simulink model "hoverSim_pid"  (R2025b)
settings: Solver=ode45  StartTime=0.0  StopTime=30  RelTol=1e-3  AbsTol=1e-3  EnableMultiTasking=on
values from neighbouring files (symbols this model uses):
  A = [0 0 0 1 0 0 ... (first row only)    [setupHover.m]    (also in setupVerdier.mat = [0 0 0 0 0 0 0 0 0 0 0 0 ... (36 elements, 6x6)])
  B = [0     0     0     0 ... (first row only)    [setupHover.m]    (also in setupVerdier.mat = [0 0 0 -0.0325954333483 0.423483129605 0 0 0 0 -0.0325954333)
  C = [1 0 0 0 0 0 ... (first row only)    [setupHover.m]    (also in setupVerdier.mat = [1 0 0 0 1 0 0 0 1 0 0 0 ... (18 elements, 3x6)])
  CMD_RATE_LIMIT = 60 * pi/180    (= 1.0471975512)    [setupHover.m]    (also in setupVerdier.mat)
  D = zeros(3,4)    [setupHover.m]    (also in setupVerdier.mat = [0  0  0  0; 0  0  0  0; 0  0  0  0])
  K = [ 1  1  0 ... (first row only)    [setupHover.m]    (also in setupVerdier.mat = [-111.8 -111.8 111.8 111.8 132.3 -132.3 0 0 0 0 132.3 -132.3)
  V_bias = 2.0    (= 2)    [setupHover.m]    (also in setupVerdier.mat)
  VMAX_AMP = 24    [setupHover.m]    (also in setupVerdier.mat)
  wcf = 2 * pi * 20    (= 125.663706144)    [setupHover.m]    (also in setupVerdier.mat)
  zetaf = 0.6    [setupHover.m]    (also in setupVerdier.mat)
undefined symbols (not defined in the file or in its folder): X, Y, Z
libraries: sm_lib x30, simulink_extras x19, nesl_utility x4, simulink x1
(part 1 of 2)
settings Model: Creator=2922887  LastModifiedBy=oleruus
settings SolverCC: AutoScaleAbsTol=off  AlgebraicLoopSolver=TrustRegion
settings DataIOCC: LimitDataPoints=on  MaxDataPoints=10000
settings OptimizationCC: LifeSpan=inf
settings DebuggingCC: UnconnectedInputMsg=warning  UnconnectedOutputMsg=warning  UnconnectedLineMsg=warning  AllowSymbolicDim=off  SFUnexpectedBacktrackingDiag=warning  SFNoUnconditionalDefaultTransitionDiag=warning  SFExecutionAtInitializationDiag=none  ArithmeticOperatorsInVariantConditions=warning
settings ModelReferenceCC: EnableRefExpFcnMdlSchedulingChecks=on
settings SFSimCC: SimUseLocalCustomCode=off  CustomCodeUndefinedFunction=UseInterfaceOnly
settings RTWCC: RTWUseLocalCustomCode=off  GPUComputeCapability=3.5  DLArmComputeVersion=19.05
settings CodeAppCC: StateflowObjectComments=on
settings GRTTargetCC: TargetLangStandard=C89/C90 (ANSI)
settings ConfigComp: CovMetricSettings=dw  CovSaveCumulativeToWorkspaceVar=on  CovSaveSingleToWorkspaceVar=on  CovExternalEMLEnable=off  CovSFcnEnable=off
settings SimscapeCC: SimscapeLogType=all  SimscapeLogSimulationStatistics=on  SimscapeLogDataHistory=10000.0
settings ExplorerConfigSet: InternalSimMechanicsExplorerSettings="<ExplorerConfiguration><canonicalview>default</canonicalview><AnimationSetting><BasePlaybackSpeed>1.0</BasePlaybackSpeed><PlaybackSpeedFactor>1.0</PlaybackSpeedFactor></AnimationSetting><TilePanel><TileInfo><Tiles Columns=\"1\" Count=\"1\" Rows=\"1\"><Column Weight=\"1\"/><Row Weight=\"1\"/><Tile Height=\"1\" Width=\"1\" X=\"0\" Y=\"0\"/></Tiles></TileInfo><SceneInfo><SceneViewer><BGColor><R>1</R><G>1</G><B>1</B></BGColor><Camera><DoPerspective>off</DoPerspective><Position><X>-0.474872206876914782</X><Y>-0.66192885214412267</Y><Z>0.674687949495536343</Z></Position><Center><X>0.0282179779907451508</X><Y>0.0797842513243843532</Y><Z>0.231109390462924141</Z></Center><Up><X>0.245225672410919443</X><Y>0.369652493337906174</Y><Z>0.896226201223598418</Z></Up><ViewLimDist>1</ViewLimDist><YLim>0.878174162375433998</YLim><XLim>0.626410921284865863</XLim></Camera></SceneViewer></SceneInfo></TilePanel><MechEditorPanel><Cameras/><GfxPanelCameraMap/><VideoCreator><PlaybackSpeedRatio>1.0</PlaybackSpeedRatio><FrameRate>30</FrameRate><VideoFormat>Motion JPEG AVI</VideoFormat><FrameSize>auto</FrameSize></VideoCreator></MechEditorPanel></ExplorerConfiguration>"

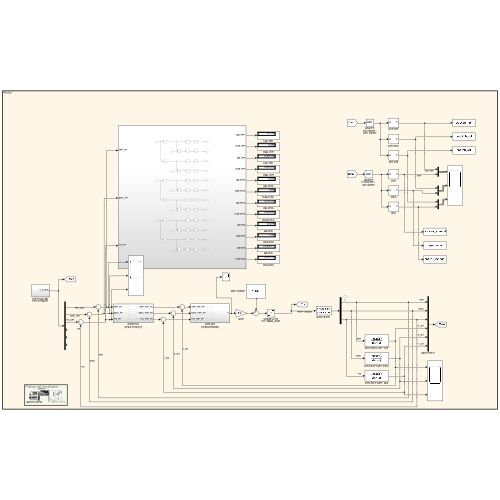
[thumbnail: Simulink's stored preview of the top-level diagram]
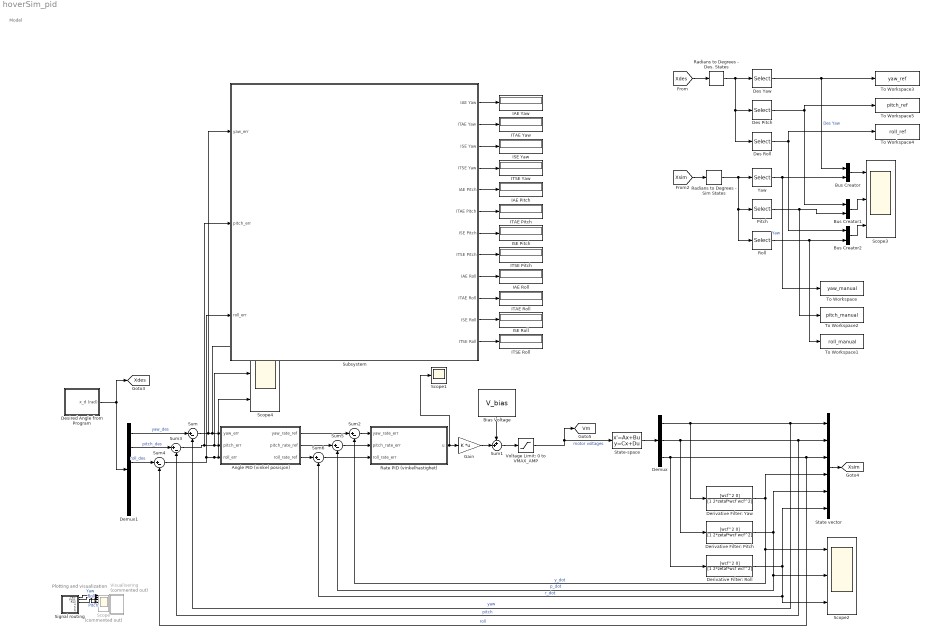
== system hoverSim_pid ==
  note: Plotting and visualization
  note: Model
  Angle PID (vinkel posisjon) : Subsystem
  Bias Voltage : Constant  Value=V_bias
  Bus Creator : BusCreator  Inputs=2
  Bus Creator1 : BusCreator  Inputs=2
  Bus Creator2 : BusCreator  Inputs=2
  Demux : Demux  Outputs=3
  Demux1 : Demux  Outputs=6
  Derivative Filter: Pitch : TransferFcn  Numerator=[wcf^2 0]  Denominator=[1 2*zetaf*wcf wcf^2]
  Derivative Filter: Roll : TransferFcn  Numerator=[wcf^2 0]  Denominator=[1 2*zetaf*wcf wcf^2]
  Derivative Filter: Yaw : TransferFcn  Numerator=[wcf^2 0]  Denominator=[1 2*zetaf*wcf wcf^2]
  Des Pitch : Selector  InputPortWidth=6  IndexOptions=Index vector (dialog)  Indices=2  OutputSizes=1
  Des Roll : Selector  InputPortWidth=6  IndexOptions=Index vector (dialog)  Indices=3  OutputSizes=1
  Des Yaw : Selector  InputPortWidth=6  IndexOptions=Index vector (dialog)  Indices=1  OutputSizes=1
  Desired Angle from Program : Subsystem
  Gain : Gain  Gain=K  Multiplication=Matrix(K*u)
  IAE Pitch : Display
  IAE Roll : Display
  IAE Yaw : Display
  ISE Pitch : Display
  ISE Roll : Display
  ISE Yaw : Display
  ITAE Pitch : Display
  ITAE Roll : Display
  ITAE Yaw : Display
  ITSE Pitch : Display
  ITSE Roll : Display
  ITSE Yaw : Display
  Pitch : Selector  InputPortWidth=6  IndexOptions=Index vector (dialog)  Indices=2  OutputSizes=1
  Radians to Degrees - Des. States : simulink_extras/Transformations/Radians to Degrees
  Radians to Degrees - Sim States : simulink_extras/Transformations/Radians to Degrees
  Rate PID (vinkelhastighet) : Subsystem
  Roll : Selector  InputPortWidth=6  IndexOptions=Index vector (dialog)  Indices=3  OutputSizes=1
  Scope : Scope  Commented=on  NumInputPorts=8
      settings: TimeSpan=30  Title=Yaw angle  ActiveDisplayYMinimum=-0.13556328685878161  ActiveDisplayYMaximum=1.2200695817290348  YLabel=deg  DataLoggingMaxPoints=10000  DataLoggingVariableName=simulationOutput
  Scope1 : Scope
      settings: ActiveDisplayYMinimum=-981.01331682218438  ActiveDisplayYMaximum=1141.4224649805096
  Scope2 : Scope  NumInputPorts=3
      settings: ActiveDisplayYMinimum=-0.50081800652745567  ActiveDisplayYMaximum=0.50362688913760034
  Scope3 : Scope  NumInputPorts=3
      settings: ActiveDisplayString=3  Title=Roll  ActiveDisplayYMinimum=-0.12798954340312932  ActiveDisplayYMaximum=1.1519058906281641  YLabel=Deg  DataLoggingVariableName=ScopeData2
  Scope4 : Scope  NumInputPorts=3
      settings: ActiveDisplayString=3  Title=Roll  ActiveDisplayYMinimum=-0.0024405494877172713  ActiveDisplayYMaximum=0.017790755348184792  YLabel=Deg  DataLoggingVariableName=ScopeData3
  Signal routing : Subsystem
  State vector : Mux  Inputs=6
  State-space : StateSpace  A=A  B=B  C=C  D=D  InitialCondition=0
  Subsystem : Subsystem
  Sum{,2..6} (6 alike) : Sum  Inputs=|+-
  Sum1 : Sum  Inputs=++|
  To Workspace : ToWorkspace  VariableName=yaw_manual  SaveFormat=Timeseries  SampleTime=-1
  To Workspace1 : ToWorkspace  VariableName=roll_manual  SaveFormat=Timeseries  SampleTime=-1
  To Workspace2 : ToWorkspace  VariableName=pitch_manual  SaveFormat=Timeseries  SampleTime=-1
  To Workspace3 : ToWorkspace  VariableName=yaw_ref  SaveFormat=Timeseries  SampleTime=-1
  To Workspace4 : ToWorkspace  VariableName=roll_ref  SaveFormat=Timeseries  SampleTime=-1
  To Workspace5 : ToWorkspace  VariableName=pitch_ref  SaveFormat=Timeseries  SampleTime=-1
  Visualisering : Subsystem  Commented=on  mask{visualization=Visualization off, PacingRate=1}
      mask prompts: PacingRate "Simulation ratio (1:x) time vs real time"
      mask TypeOptions visualization: Visualization  on | Visualization off
      mask Callback visualization:
      | if get_param(append(bdroot,'/Visualisering'),'visualization') == 'Visualization  on'
      |    set_param(bdroot,'EnablePacing','on')
      | elseif get_param(append(bdroot,'/Visualisering'),'visualization') == 'Visualization off'
      |    set_param(bdroot,'EnablePacing','off')
      | end
      mask Callback PacingRate:
      | temp_param = str2num(get_param(append(bdroot,'/Visualisering'),'PacingRate'));
      | if temp_param >= 0.003 && temp_param < 0.0078
      |     set_param(bdroot,'PacingRate','0.0039')
      |     set_param(append(bdroot,'/Visualisering'),'PacingRate','0.0039')
      | elseif temp_param >= 0.0078 && temp_param < 0.0156
      |     set_param(bdroot,'PacingRate','0.0078')
      |     set_param(append(bdroot,'/Visualisering'),'PacingRate','0.0078')
      | elseif temp_param >= 0.0156 && temp_param < 0.0313
      |     set_param(bdroot,'PacingRate','0.0156')
      |     set_param(append(bdroot,'/Visualisering'),'PacingRate','0.0156')
      | elseif temp_param >= 0.0313 && temp_param < 0.0625
      |     set_param(bdroot,'PacingRate','0.0313')
      |     set_param(append(bdroot,'/Visualisering'),'PacingRate','0.0313')
      | elseif temp_param >= 0.0625 && temp_param < 0.1250
      |     set_param(bdroot,'PacingRate','0.0625')
      |     set_param(append(bdroot,'/Visualisering'),'PacingRate','0.0625')
      | elseif temp_param >= 0.1250 && temp_param < 0.2500
      |     set_param(bdroot,'PacingRate','0.1250')
      |     set_param(append(bdroot,'/Visualisering'),'PacingRate','0.1250')
      | elseif temp_param >= 0.2500 && temp_param < 0.5000
      |     set_param(bdroot, 'PacingRate','0.2500')
      |     set_param(append(bdroot,'/Visualisering'),'PacingRate','0.2500')
      | elseif temp_param >= 0.5000 && temp_param < 1
      |     set_param(bdroot, 'PacingRate','0.5000')
      |     set_param(append(bdroot,'/Visualisering'),'PacingRate','0.5000')
      | elseif temp_param >= 1 && temp_param < 2
      |     set_param(bdroot, 'PacingRate','1')
      |     set_param(append(bdroot,'/Visualisering'),'PacingRate','1')
      | elseif temp_param >= 2 && temp_param < 4
      |     set_param(bdroot, 'PacingRate','2')
      |     set_param(append(bdroot,'/Visualisering'),'PacingRate','2')
      | elseif temp_param >= 4 && temp_param < 8
      |     set_param(bdroot, 'PacingRate','4')
      |     set_param(append(bdroot,'/Visualisering'),'PacingRate','4')
      | elseif temp_param >= 8 && temp_param < 16
      |     set_param(bdroot, 'PacingRate','8')
      |     set_param(append(bdroot,'/Visualisering'),'PacingRate','8')
      | elseif temp_param >= 16 && temp_param < 32
      |     set_param(bdroot, 'PacingRate','16')
      |     set_param(append(bdroot,'/Visualisering'),'PacingRate','16')
      | elseif temp_param >= 32 && temp_param < 64
      |     set_param(bdroot, 'PacingRate','32')
      |     set_param(append(bdroot,'/Visualisering'),'PacingRate','32')
      | elseif temp_param >= 64 && temp_param < 128
      |     set_param(bdroot, 'PacingRate','64')
      |     set_param(append(bdroot,'/Visualisering'),'PacingRate','64')
      | elseif temp_param >= 128 && temp_param < 256
      |     set_param(bdroot, 'PacingRate','128')
      |     set_param(append(bdroot,'/Visualisering'),'PacingRate','128')
      | elseif temp_param >= 256
      |     set_param(bdroot, 'PacingRate','256')
      |     set_param(append(bdroot,'/Visualisering'),'PacingRate','256')
      | end
      mask DialogControl Control2 Prompt: For a 1:1 relation between the visualization model and the plotted data, the simulation ratio in this box should match the ratio in the Mechanics Explorer.
      mask DialogControl x256x Prompt: 0.0039 = 1/256x
      mask DialogControl x128x Prompt: 0.0078 = 1/128x
      mask DialogControl x64x Prompt: 0.0156 = 1/64x
      mask DialogControl x32x Prompt: 0.0313 = 1/32x
      mask DialogControl x16x Prompt: 0.0625 = 1/16x
      mask DialogControl x8x Prompt: 0.1250 = 1/8x
      mask DialogControl x4x Prompt: 0.2500 = 1/4x
      mask DialogControl x2x Prompt: 0.5000 = 1/2x
      mask Display: image('$imagefile'); % Use "Edit Image" on toolstrip to change.
  Voltage Limit: 0 to VMAX_AMP : Saturate  UpperLimit=VMAX_AMP  LowerLimit=0  LinearizeAsGain=off
  Yaw : Selector  InputPortWidth=6  IndexOptions=Index vector (dialog)  Indices=1  OutputSizes=1
  tag scope: Vm=global, Xdes=global, Xsim=global
  wires:
  Gain/1 -> Sum1/2
  Voltage Limit: 0 to VMAX_AMP/1 -> [Vm], State-space/1  "motor voltages"
  Derivative Filter: Roll/1 -> Scope2/3, Sum6/2, State vector/6  "r_dot"
  Derivative Filter: Yaw/1 -> Sum2/2, Scope2/1, State vector/4  "y_dot"
  State-space/1 -> Demux/1
  State vector/1 -> [Xsim]
  Demux/1 -> Derivative Filter: Yaw/1, Sum/2, State vector/1  "yaw"
  Sum1/1 -> Voltage Limit: 0 to VMAX_AMP/1
  Bias Voltage/1 -> Sum1/1
  Demux/2 -> Derivative Filter: Pitch/1, State vector/2, Sum3/2  "pitch"
  Derivative Filter: Pitch/1 -> Scope2/2, Sum5/2, State vector/5  "p_dot"
  Demux/3 -> State vector/3, Sum4/2, Derivative Filter: Roll/1  "roll"
  Signal routing/1(Yaw) -> Scope/1  "Yaw"
  Signal routing/2(Pitch) -> Scope/4, Scope/2  "Pitch"
  Signal routing/3(Roll) -> Scope/3  "Roll"
  Desired Angle from Program/1(x_d (rad)) -> Demux1/1, [Xdes]
  Sum2/1 -> Rate PID (vinkelhastighet)/1(yaw_rate_err)
  Demux1/1 -> Sum/1  "yaw_des"
  Sum/1 -> Subsystem/1(yaw_err), Scope4/1, Angle PID (vinkel posisjon)/1(yaw_err)
  Demux1/2 -> Sum3/1  "pitch_des"
  Demux1/3 -> Sum4/1  "roll_des"
  Sum3/1 -> Subsystem/2(pitch_err), Scope4/2, Angle PID (vinkel posisjon)/2(pitch_err)
  Sum4/1 -> Subsystem/3(roll_err), Scope4/3, Angle PID (vinkel posisjon)/3(roll_err)
  Rate PID (vinkelhastighet)/1(u) -> Scope1/1, Gain/1
  Sum5/1 -> Rate PID (vinkelhastighet)/2(pitch_rate_err)
  Sum6/1 -> Rate PID (vinkelhastighet)/3(roll_rate_err)
  Angle PID (vinkel posisjon)/1(yaw_rate_ref) -> Sum2/1
  Angle PID (vinkel posisjon)/2(pitch_rate_ref) -> Sum5/1
  Angle PID (vinkel posisjon)/3(roll_rate_ref) -> Sum6/1
  Des Pitch/1 -> Bus Creator1/1, To Workspace5/1
  Pitch/1 -> To Workspace2/1, Bus Creator1/2
  Yaw/1 -> To Workspace/1, Bus Creator/2  "Yaw"
  Des Roll/1 -> Bus Creator2/1, To Workspace4/1
  Des Yaw/1 -> Bus Creator/1, To Workspace3/1  "Des Yaw"
  Radians to Degrees - Sim States/1 -> Roll/1, Pitch/1, Yaw/1
  [Xsim] -> Radians to Degrees - Sim States/1
  [Xdes] -> Radians to Degrees - Des. States/1
  Radians to Degrees - Des. States/1 -> Des Roll/1, Des Pitch/1, Des Yaw/1
  Roll/1 -> To Workspace1/1, Bus Creator2/2
  Bus Creator/1 -> Scope3/1
  Bus Creator1/1 -> Scope3/2
  Bus Creator2/1 -> Scope3/3
  Subsystem/10(ITAE Roll) -> ITAE Roll/1
  Subsystem/9(IAE Roll) -> IAE Roll/1
  Subsystem/1("IAE Yaw ") -> IAE Yaw/1
  Subsystem/2(ITAE Yaw) -> ITAE Yaw/1
  Subsystem/5(IAE Pitch) -> IAE Pitch/1
  Subsystem/6(ITAE Pitch) -> ITAE Pitch/1
  Subsystem/3(ISE Yaw) -> ISE Yaw/1
  Subsystem/4(ITSE Yaw) -> ITSE Yaw/1
  Subsystem/7(ISE Pitch) -> ISE Pitch/1
  Subsystem/8(ITSE Pitch) -> ITSE Pitch/1
  Subsystem/11(ISE Roll) -> ISE Roll/1
  Subsystem/12(ITSE Roll) -> ITSE Roll/1

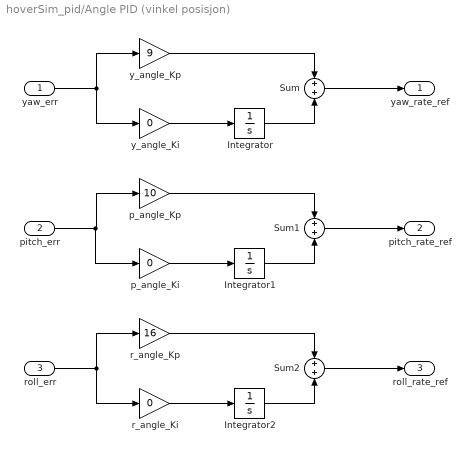
== system hoverSim_pid/Angle PID (vinkel posisjon) ==
  yaw_err : Inport
  pitch_err : Inport  Port=2
  roll_err : Inport  Port=3
  Integrator : Integrator
  Integrator1 : Integrator
  Integrator2 : Integrator
  Sum : Sum  Inputs=+|+
  Sum1 : Sum  Inputs=+|+
  Sum2 : Sum  Inputs=+|+
  p_angle_Ki : Gain  Gain=0
  p_angle_Kp : Gain  Gain=10
  r_angle_Ki : Gain  Gain=0
  r_angle_Kp : Gain  Gain=16
  y_angle_Ki : Gain  Gain=0
  y_angle_Kp : Gain  Gain=9
  yaw_rate_ref : Outport
  pitch_rate_ref : Outport  Port=2
  roll_rate_ref : Outport  Port=3
  wires:
  Sum/1 -> yaw_rate_ref/1
  pitch_err/1 -> p_angle_Ki/1, p_angle_Kp/1
  p_angle_Ki/1 -> Integrator1/1
  Integrator1/1 -> Sum1/2
  p_angle_Kp/1 -> Sum1/1
  y_angle_Kp/1 -> Sum/1
  Integrator/1 -> Sum/2
  y_angle_Ki/1 -> Integrator/1
  yaw_err/1 -> y_angle_Ki/1, y_angle_Kp/1
  Sum1/1 -> pitch_rate_ref/1
  roll_err/1 -> r_angle_Kp/1, r_angle_Ki/1
  r_angle_Kp/1 -> Sum2/1
  r_angle_Ki/1 -> Integrator2/1
  Integrator2/1 -> Sum2/2
  Sum2/1 -> roll_rate_ref/1

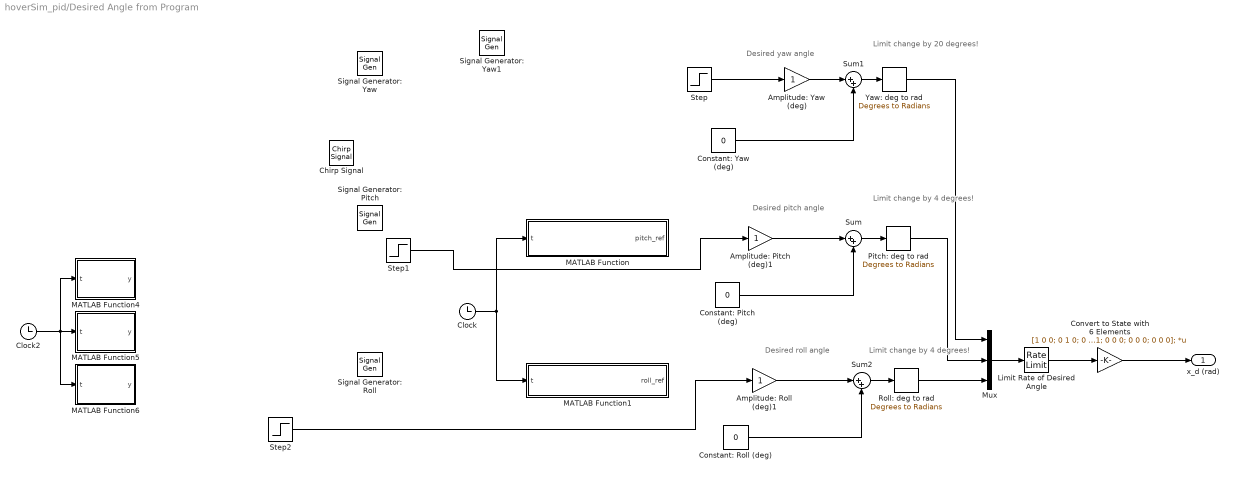
== system hoverSim_pid/Desired Angle from Program ==
  note: Limit change by
      | 4 degrees!
  note: Limit change by
      | 20 degrees!
  note: Limit change by
      | 4 degrees!
  note: Desired roll angle
  note: Desired pitch angle
  note: Desired yaw angle
  Amplitude: Pitch (deg)1 : Gain
  Amplitude: Roll (deg)1 : Gain
  Amplitude: Yaw (deg) : Gain
  Chirp Signal : simulink/Sources/Chirp Signal  f1=0.1  T=30  f2=0.7
  Clock : Clock
  Clock2 : Clock
  Constant: Pitch (deg) : Constant  Value=0
  Constant: Roll (deg) : Constant  Value=0
  Constant: Yaw (deg) : Constant  Value=0
  Convert to State with 6 Elements : Gain  Gain=[1 0 0; 0 1 0; 0 0 1; 0 0 0; 0 0 0; 0 0 0];  Multiplication=Matrix(K*u)
  Limit Rate of Desired Angle : RateLimiter  RisingSlewLimit=CMD_RATE_LIMIT  FallingSlewLimit=-CMD_RATE_LIMIT
  MATLAB Function : MATLAB Function  TreatAsAtomicUnit=on
  MATLAB Function1 : MATLAB Function  TreatAsAtomicUnit=on
  MATLAB Function4 : MATLAB Function  TreatAsAtomicUnit=on
  MATLAB Function5 : MATLAB Function  TreatAsAtomicUnit=on
  MATLAB Function6 : MATLAB Function  TreatAsAtomicUnit=on
  Mux : Mux  Inputs=3
  Pitch: deg to rad : simulink_extras/Transformations/Degrees to Radians
  Roll: deg to rad : simulink_extras/Transformations/Degrees to Radians
  Signal Generator: Pitch : SignalGenerator  WaveForm=square  Frequency=0.1
  Signal Generator: Roll : SignalGenerator  WaveForm=square  Frequency=0.08
  Signal Generator: Yaw : SignalGenerator  WaveForm=square  Frequency=0.04
  Signal Generator: Yaw1 : SignalGenerator  WaveForm=square  Frequency=0.06
  Step : Step  Time=2  SampleTime=0
  Step1 : Step  Time=5  SampleTime=0
  Step2 : Step  Time=8  SampleTime=0
  Sum : Sum  Inputs=|++
  Sum1 : Sum  Inputs=|++
  Sum2 : Sum  Inputs=|++
  Yaw: deg to rad : simulink_extras/Transformations/Degrees to Radians
  x_d (rad) : Outport
  wires:
  Convert to State with 6 Elements/1 -> x_d (rad)/1
  Limit Rate of Desired Angle/1 -> Convert to State with 6 Elements/1
  Roll: deg to rad/1 -> Mux/3
  Pitch: deg to rad/1 -> Mux/2
  Yaw: deg to rad/1 -> Mux/1
  Sum2/1 -> Roll: deg to rad/1
  Amplitude: Roll (deg)1/1 -> Sum2/1
  Constant: Roll (deg)/1 -> Sum2/2
  Sum/1 -> Pitch: deg to rad/1
  Amplitude: Pitch (deg)1/1 -> Sum/1
  Constant: Pitch (deg)/1 -> Sum/2
  Sum1/1 -> Yaw: deg to rad/1
  Amplitude: Yaw (deg)/1 -> Sum1/1
  Constant: Yaw (deg)/1 -> Sum1/2
  Mux/1 -> Limit Rate of Desired Angle/1
  Clock/1 -> MATLAB Function/1(t), MATLAB Function1/1(t)
  Clock2/1 -> MATLAB Function6/1(t), MATLAB Function4/1(t), MATLAB Function5/1(t)
  Step/1 -> Amplitude: Yaw (deg)/1
  Step1/1 -> Amplitude: Pitch (deg)1/1
  Step2/1 -> Amplitude: Roll (deg)1/1

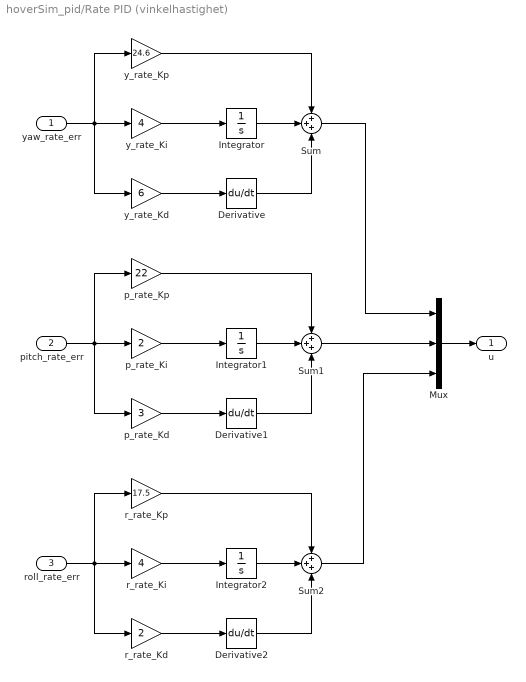
== system hoverSim_pid/Rate PID (vinkelhastighet) ==
  yaw_rate_err : Inport
  pitch_rate_err : Inport  Port=2
  roll_rate_err : Inport  Port=3
  Derivative : Derivative
  Derivative1 : Derivative
  Derivative2 : Derivative
  Integrator : Integrator
  Integrator1 : Integrator
  Integrator2 : Integrator
  Mux : Mux  Inputs=3
  Sum : Sum  Inputs=+++
  Sum1 : Sum  Inputs=+++
  Sum2 : Sum  Inputs=+++
  p_rate_Kd : Gain  Gain=3
  p_rate_Ki : Gain  Gain=2
  p_rate_Kp : Gain  Gain=22
  r_rate_Kd : Gain  Gain=2
  r_rate_Ki : Gain  Gain=4
  r_rate_Kp : Gain  Gain=17.5
  y_rate_Kd : Gain  Gain=6
  y_rate_Ki : Gain  Gain=4
  y_rate_Kp : Gain  Gain=24.6
  u : Outport
  wires:
  Mux/1 -> u/1
  y_rate_Ki/1 -> Integrator/1
  y_rate_Kd/1 -> Derivative/1
  Integrator/1 -> Sum/2
  y_rate_Kp/1 -> Sum/1
  Derivative/1 -> Sum/3
  yaw_rate_err/1 -> y_rate_Kd/1, y_rate_Kp/1, y_rate_Ki/1
  p_rate_Ki/1 -> Integrator1/1
  p_rate_Kp/1 -> Sum1/1
  pitch_rate_err/1 -> p_rate_Kd/1, p_rate_Kp/1, p_rate_Ki/1
  Integrator1/1 -> Sum1/2
  p_rate_Kd/1 -> Derivative1/1
  Derivative1/1 -> Sum1/3
  r_rate_Ki/1 -> Integrator2/1
  r_rate_Kp/1 -> Sum2/1
  roll_rate_err/1 -> r_rate_Kd/1, r_rate_Kp/1, r_rate_Ki/1
  Integrator2/1 -> Sum2/2
  r_rate_Kd/1 -> Derivative2/1
  Derivative2/1 -> Sum2/3
  Sum/1 -> Mux/1
  Sum2/1 -> Mux/3
  Sum1/1 -> Mux/2

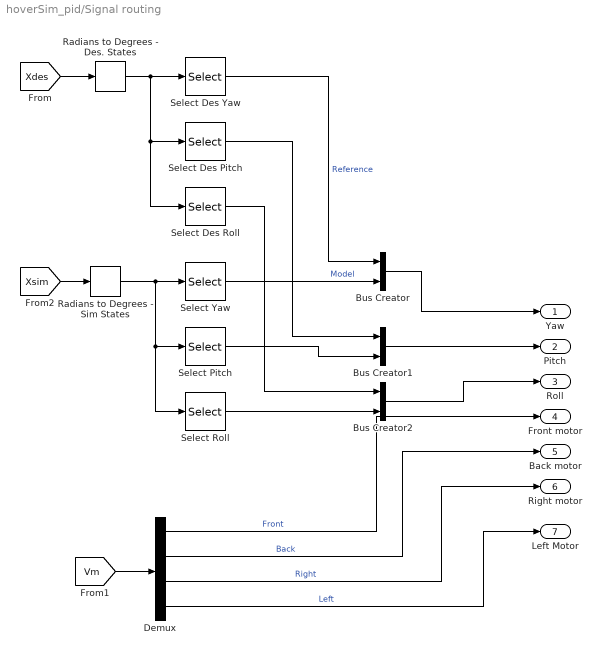
== system hoverSim_pid/Signal routing ==
  Bus Creator : BusCreator  Inputs=2
  Bus Creator1 : BusCreator  Inputs=2
  Bus Creator2 : BusCreator  Inputs=2
  Demux : Demux
  Radians to Degrees - Des. States : simulink_extras/Transformations/Radians to Degrees
  Radians to Degrees - Sim States : simulink_extras/Transformations/Radians to Degrees
  Select Des Pitch : Selector  InputPortWidth=6  IndexOptions=Index vector (dialog)  Indices=2  OutputSizes=1
  Select Des Roll : Selector  InputPortWidth=6  IndexOptions=Index vector (dialog)  Indices=3  OutputSizes=1
  Select Des Yaw : Selector  InputPortWidth=6  IndexOptions=Index vector (dialog)  Indices=1  OutputSizes=1
  Select Pitch : Selector  InputPortWidth=6  IndexOptions=Index vector (dialog)  Indices=2  OutputSizes=1
  Select Roll : Selector  InputPortWidth=6  IndexOptions=Index vector (dialog)  Indices=3  OutputSizes=1
  Select Yaw : Selector  InputPortWidth=6  IndexOptions=Index vector (dialog)  Indices=1  OutputSizes=1
  Yaw : Outport
  Pitch : Outport  Port=2
  Roll : Outport  Port=3
  Front motor : Outport  Port=4
  Back motor : Outport  Port=5
  Right motor : Outport  Port=6
  Left Motor : Outport  Port=7
  wires:
  Select Des Roll/1 -> Bus Creator2/1
  Select Des Pitch/1 -> Bus Creator1/1
  Select Des Yaw/1 -> Bus Creator/1  "Reference"
  Radians to Degrees - Des. States/1 -> Select Des Roll/1, Select Des Pitch/1, Select Des Yaw/1
  Select Roll/1 -> Bus Creator2/2
  Select Pitch/1 -> Bus Creator1/2
  Select Yaw/1 -> Bus Creator/2  "Model"
  Bus Creator2/1 -> Roll/1
  Radians to Degrees - Sim States/1 -> Select Roll/1, Select Pitch/1, Select Yaw/1
  Bus Creator1/1 -> Pitch/1
  Bus Creator/1 -> Yaw/1
  [Xsim] -> Radians to Degrees - Sim States/1
  [Xdes] -> Radians to Degrees - Des. States/1
  [Vm] -> Demux/1
  Demux/1 -> Front motor/1  "Front"
  Demux/2 -> Back motor/1  "Back"
  Demux/3 -> Right motor/1  "Right"
  Demux/4 -> Left Motor/1  "Left"

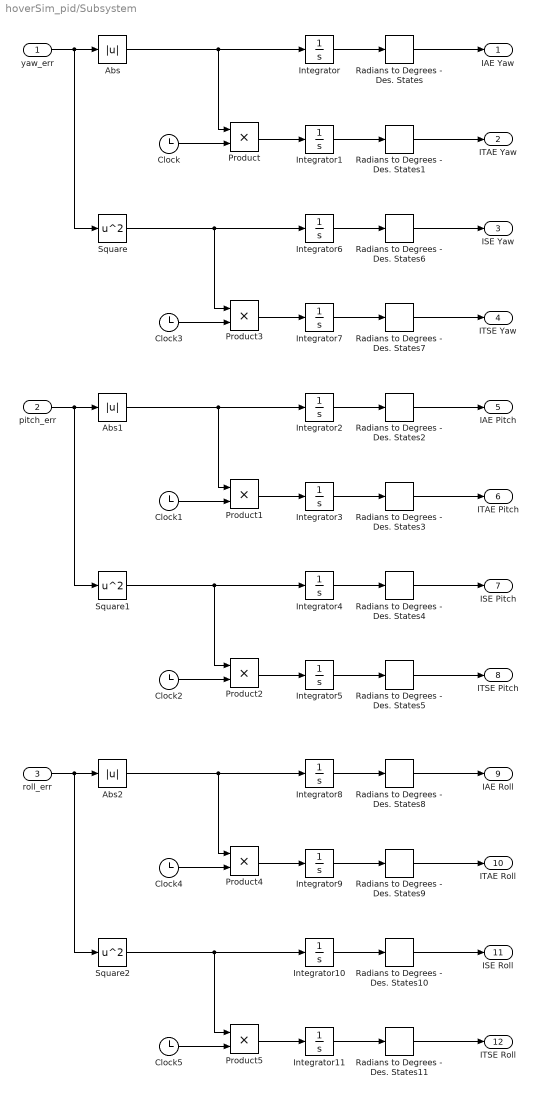
== system hoverSim_pid/Subsystem ==
  yaw_err : Inport
  pitch_err : Inport  Port=2
  roll_err : Inport  Port=3
  Abs : Abs  SaturateOnIntegerOverflow=off
  Abs1 : Abs  SaturateOnIntegerOverflow=off
  Abs2 : Abs  SaturateOnIntegerOverflow=off
  Clock{,1..5} (6 alike) : Clock
  Integrator{,1..11} (12 alike) : Integrator
  Product{,1..5} (6 alike) : Product
  Radians to Degrees - Des. States{,1..11} (12 alike) : simulink_extras/Transformations/Radians to Degrees
  Square : Math  Operator=square
  Square1 : Math  Operator=square
  Square2 : Math  Operator=square
  "IAE Yaw " : Outport
  ITAE Yaw : Outport  Port=2
  ISE Yaw : Outport  Port=3
  ITSE Yaw : Outport  Port=4
  IAE Pitch : Outport  Port=5
  ITAE Pitch : Outport  Port=6
  ISE Pitch : Outport  Port=7
  ITSE Pitch : Outport  Port=8
  IAE Roll : Outport  Port=9
  ITAE Roll : Outport  Port=10
  ISE Roll : Outport  Port=11
  ITSE Roll : Outport  Port=12
  wires:
  yaw_err/1 -> Abs/1, Square/1
  Clock/1 -> Product/2
  Abs/1 -> Integrator/1, Product/1
  Product/1 -> Integrator1/1
  Integrator/1 -> Radians to Degrees - Des. States/1
  Integrator1/1 -> Radians to Degrees - Des. States1/1
  Square/1 -> Product3/1, Integrator6/1
  Clock3/1 -> Product3/2
  Product3/1 -> Integrator7/1
  Integrator7/1 -> Radians to Degrees - Des. States7/1
  Integrator6/1 -> Radians to Degrees - Des. States6/1
  Radians to Degrees - Des. States/1 -> "IAE Yaw "/1
  Radians to Degrees - Des. States1/1 -> ITAE Yaw/1
  Radians to Degrees - Des. States6/1 -> ISE Yaw/1
  Radians to Degrees - Des. States7/1 -> ITSE Yaw/1
  Clock1/1 -> Product1/2
  Radians to Degrees - Des. States5/1 -> ITSE Pitch/1
  Clock2/1 -> Product2/2
  Product1/1 -> Integrator3/1
  Integrator3/1 -> Radians to Degrees - Des. States3/1
  Abs1/1 -> Integrator2/1, Product1/1
  Integrator2/1 -> Radians to Degrees - Des. States2/1
  pitch_err/1 -> Abs1/1, Square1/1
  Integrator5/1 -> Radians to Degrees - Des. States5/1
  Integrator4/1 -> Radians to Degrees - Des. States4/1
  Radians to Degrees - Des. States4/1 -> ISE Pitch/1
  Product2/1 -> Integrator5/1
  Square1/1 -> Product2/1, Integrator4/1
  Radians to Degrees - Des. States3/1 -> ITAE Pitch/1
  Radians to Degrees - Des. States2/1 -> IAE Pitch/1
  Clock4/1 -> Product4/2
  Radians to Degrees - Des. States11/1 -> ITSE Roll/1
  Clock5/1 -> Product5/2
  Product4/1 -> Integrator9/1
  Integrator9/1 -> Radians to Degrees - Des. States9/1
  Abs2/1 -> Integrator8/1, Product4/1
  Integrator8/1 -> Radians to Degrees - Des. States8/1
  roll_err/1 -> Abs2/1, Square2/1
  Integrator11/1 -> Radians to Degrees - Des. States11/1
  Integrator10/1 -> Radians to Degrees - Des. States10/1
  Radians to Degrees - Des. States10/1 -> ISE Roll/1
  Product5/1 -> Integrator11/1
  Square2/1 -> Product5/1, Integrator10/1
  Radians to Degrees - Des. States9/1 -> ITAE Roll/1
  Radians to Degrees - Des. States8/1 -> IAE Roll/1

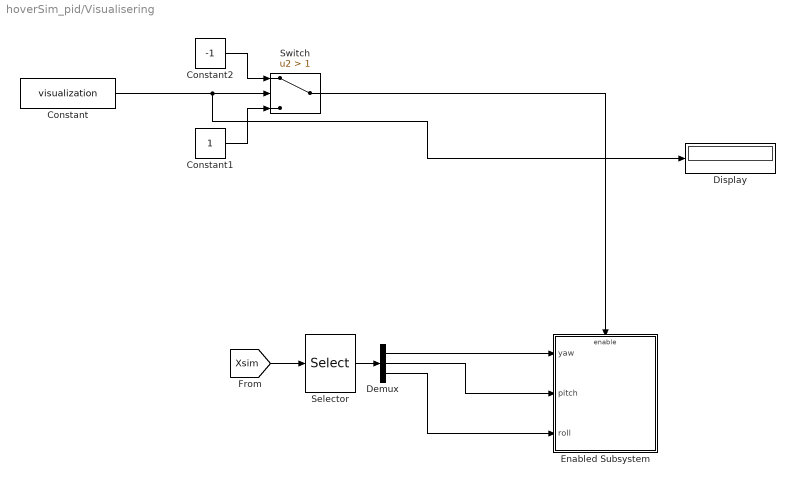
== system hoverSim_pid/Visualisering ==
  Constant : Constant  Value=visualization
  Constant1 : Constant
  Constant2 : Constant  Value=-1
  Demux : Demux  Outputs=3
  Display : Display
  Enabled Subsystem : Subsystem  TreatAsAtomicUnit=on
  Selector : Selector  InputPortWidth=6  IndexOptions=Index vector (dialog)  Indices=[1 2 3]  OutputSizes=1
  Switch : Switch  Criteria=u2 > Threshold  Threshold=1  SaturateOnIntegerOverflow=off  InputSameDT=off
  wires:
  Constant1/1 -> Switch/3
  Constant2/1 -> Switch/1
  Switch/1 -> Enabled Subsystem/Enable
  Constant/1 -> Display/1, Switch/2
  [Xsim] -> Selector/1
  Selector/1 -> Demux/1
  Demux/1 -> Enabled Subsystem/1(yaw)
  Demux/2 -> Enabled Subsystem/2(pitch)
  Demux/3 -> Enabled Subsystem/3(roll)
